simulink model "pokus07_video"  (R2023a)
settings: Solver=VariableStepAuto  StartTime=0.0  StopTime=10.0  RelTol=1e-3
undefined symbols (not defined in the file): c
libraries: Miscellaneous x840, Memory_Blocks_Lib x251, Decoders_Lib x10, simulink_extras x10, Counters_Lib x4, Bit_Multiplexers_Lib x1, Byte_Multiplexers_Lib x1
(part 1 of 5)
settings Model: Creator=Jozko Mrkvicka  LastModifiedBy=Jozko Mrkvicka

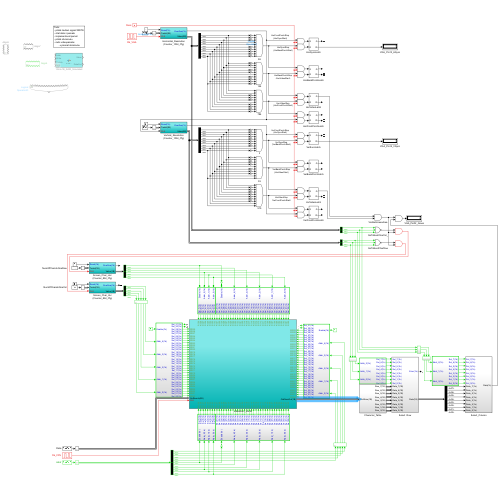
[thumbnail: Simulink's stored preview of the top-level diagram]
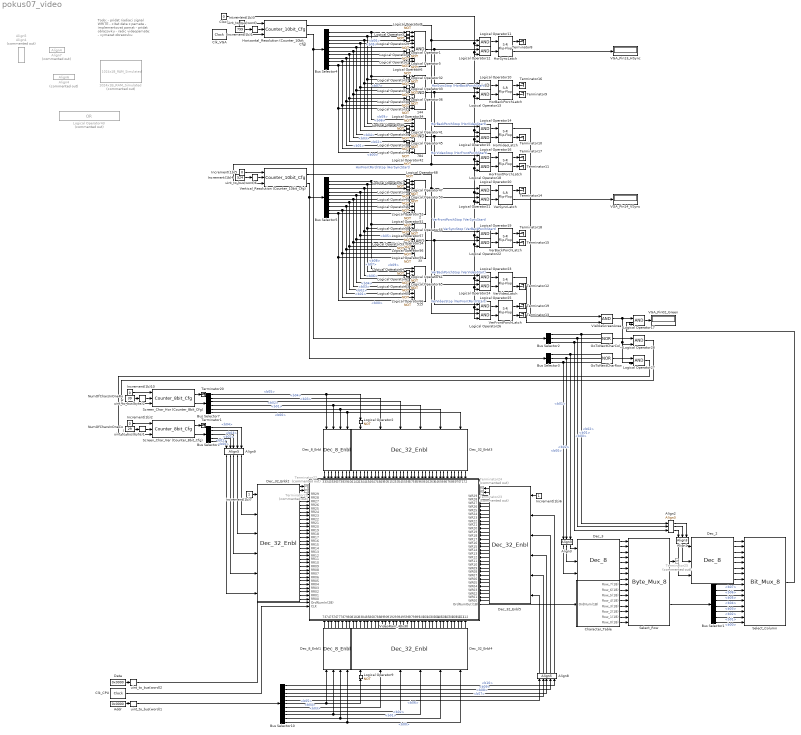
== system pokus07_video ==
  note: Todo:
      | - pridat riadiaci signal WRITE
      | - citat data z pamate
      | - implementovat pamat
      | - pridat obrazovku
      | - radic videopamate:
      | 	- vymazat obrazovku
  1024x1B_RAM_Simulated : Memory_Blocks_Lib/1024x1B_RAM_Simulated  Commented=on  SystemSampleTime=-1  VariantActivationTime=update diagram  Latency=0  AutoFrameSizeCalculation=off
  {2,35,96,144,515,784} (6 alike) : Logic  Inputs=10  IconShape=distinctive  AllPortsSameDT=off  OutDataTypeStr=boolean
  Addr : Constant  Value=0x0000  OutDataTypeStr=uint16
  Align1 : Miscellaneous/Align3  SystemSampleTime=-1  VariantActivationTime=update diagram  Latency=0  AutoFrameSizeCalculation=off
  Align2 : Miscellaneous/Align3  SystemSampleTime=-1  VariantActivationTime=update diagram  Latency=0  AutoFrameSizeCalculation=off
  Align3 : Miscellaneous/Align3  SystemSampleTime=-1  VariantActivationTime=update diagram  Latency=0  AutoFrameSizeCalculation=off
  Align4 : Miscellaneous/Align6  Commented=on
  Align5 : Miscellaneous/Align4  Commented=on
  Align7 : Miscellaneous/Align4  Commented=on
  Align8 : Miscellaneous/Align5
  Align9 : Miscellaneous/Align5
  Bus Selector1 : BusSelector  OutputSignals=b07,b06,b05,b04,b03,b02,b01,b00
  Bus Selector10 : BusSelector  OutputSignals=b10,b09,b08,b07,b06,b05,b04,b03,b02,b01,b00
  Bus Selector2 : BusSelector  OutputSignals=b02,b01,b00
  Bus Selector3 : BusSelector  OutputSignals=b02,b01,b00
  Bus Selector4 : BusSelector  OutputSignals=b09,b08,b07,b06,b05,b04,b03,b02,b01,b00
  Bus Selector5 : BusSelector  OutputSignals=b09,b08,b07,b06,b05,b04,b03,b02,b01,b00
  Bus Selector6 : BusSelector  OutputSignals=b04,b03,b02,b01,b00
  Bus Selector7 : BusSelector  OutputSignals=b05,b04,b03,b02,b01,b00
  Character_Table : Subsystem
  Clk_CPU : simulink_extras/Flip Flops/Clock  period=1
  Clk_VGA : simulink_extras/Flip Flops/Clock  period=1
  Clock : Constant  Value=0  OutDataTypeStr=uint16
  Data : Constant  Value=0x0000  OutDataTypeStr=uint16
  Dec_2 : Decoders_Lib/Dec_8  SystemSampleTime=-1  VariantActivationTime=update diagram  Latency=0  AutoFrameSizeCalculation=off
  Dec_3 : Decoders_Lib/Dec_8  SystemSampleTime=-1  VariantActivationTime=update diagram  Latency=0  AutoFrameSizeCalculation=off
  Dec_32_Enbl{2..5} (4 alike) : Decoders_Lib/Dec_32_Enbl  SystemSampleTime=-1  VariantActivationTime=update diagram  Latency=0  AutoFrameSizeCalculation=off
  Dec_8_Enbl : Decoders_Lib/Dec_8_Enbl  SystemSampleTime=-1  VariantActivationTime=update diagram  Latency=0  AutoFrameSizeCalculation=off
  Dec_8_Enbl1 : Decoders_Lib/Dec_8_Enbl  SystemSampleTime=-1  VariantActivationTime=update diagram  Latency=0  AutoFrameSizeCalculation=off
  GoToNextCharCol_ : Logic  Operator=NOR  Inputs=3  IconShape=distinctive  AllPortsSameDT=off  OutDataTypeStr=boolean
  GoToNextCharRow : Logic  Operator=NOR  Inputs=3  IconShape=distinctive  AllPortsSameDT=off  OutDataTypeStr=boolean
  HorBackPorchLatch : simulink_extras/Flip Flops/S-R Flip-Flop  initial_condition=0
  HorFrontPorchLatch : simulink_extras/Flip Flops/S-R Flip-Flop  initial_condition=0
  HorSyncLatch : simulink_extras/Flip Flops/S-R Flip-Flop  initial_condition=0
  HorVideoLatch : simulink_extras/Flip Flops/S-R Flip-Flop  initial_condition=0
  Horizontal_Resolution (Counter_10bit_Cfg) : Counters_Lib/Counter_10bit_Cfg  SystemSampleTime=-1  VariantActivationTime=update diagram  Latency=0  AutoFrameSizeCalculation=off
  Increment(1b)1 : Constant  Value=799  OutDataTypeStr=uint16
  Increment(1b){2..3,5,10} (4 alike) : Constant  Value=0  OutDataTypeStr=boolean
  Increment(1b)4 : Constant  Value=524  OutDataTypeStr=uint16
  Increment(1b)6 : Constant  OutDataTypeStr=boolean
  Increment(1b)7 : Constant  OutDataTypeStr=boolean
  Logical Operator{1..9,29..42,44..68} (48 alike) : Logic  Operator=NOT  IconShape=distinctive  AllPortsSameDT=off  OutDataTypeStr=boolean
  Logical Operator{10..28} (19 alike) : Logic  IconShape=distinctive  AllPortsSameDT=off  OutDataTypeStr=boolean
  Logical Operator43 : Logic  Commented=on  Operator=OR  Inputs=16  IconShape=distinctive  OutDataTypeStr=boolean
  "NumOfCharsInOneCol      " : Constant  Value=29  OutDataTypeStr=uint8
  "NumOfCharsInOneRow      " : Constant  Value=39  OutDataTypeStr=uint8
  Screen_Char_Hor (Counter_8bit_Cfg) : Counters_Lib/Counter_8bit_Cfg  SystemSampleTime=-1  VariantActivationTime=update diagram  Latency=0  AutoFrameSizeCalculation=off
  Screen_Char_Ver (Counter_8bit_Cfg) : Counters_Lib/Counter_8bit_Cfg  SystemSampleTime=-1  VariantActivationTime=update diagram  Latency=0  AutoFrameSizeCalculation=off
  Select_Column : Bit_Multiplexers_Lib/Bit_Mux_8  SystemSampleTime=-1  VariantActivationTime=update diagram  Latency=0  AutoFrameSizeCalculation=off
  Select_Row : Byte_Multiplexers_Lib/Byte_Mux_8  SystemSampleTime=-1  VariantActivationTime=update diagram  Latency=0  AutoFrameSizeCalculation=off
  Terminator{1,8..20} (14 alike) : Terminator
  Terminator{21..25} (5 alike) : Terminator  Commented=on
  VGA_Pin02_Green : Display
  VGA_Pin13_HSync : Display
  VGA_Pin14_VSync : Display
  VerBackPorchLatch : simulink_extras/Flip Flops/S-R Flip-Flop  initial_condition=0
  VerFrontPorchLatch : simulink_extras/Flip Flops/S-R Flip-Flop  initial_condition=0
  VerSyncLatch : simulink_extras/Flip Flops/S-R Flip-Flop  initial_condition=0
  VerVideoLatch : simulink_extras/Flip Flops/S-R Flip-Flop  initial_condition=0
  Vertical_Resolution (Counter_10bit_Cfg) : Counters_Lib/Counter_10bit_Cfg  SystemSampleTime=-1  VariantActivationTime=update diagram  Latency=0  AutoFrameSizeCalculation=off
  VideoRam_40x30 : Subsystem
      settings: PortSchema="{\"entries\":[{\"content\":{\"sides\":[{\"content\":{\"connectorIds\":[\"In1\",\"In2\",\"In3\",\"In4\",\"In5\",\"In6\",\"In7\",\"In8\",\"In9\",\"In10\",\"In11\",\"In12\",\"In13\",\"In14\",\"In15\",\"In16\",\"In17\",\"In18\",\"In19\",\"In20\",\"In21\",\"In22\",\"In23\",\"In24\",\"In25\",\"In26\",\"In27\",\"In28\",\"In29\",\"In30\",\"In31\",\"In32\"]},\"type\":\"ConnectorPlacement.EquallySpacedRectSide\",\"uuid\":\"d52aabea-5fd3-45ae-978c-84320c8647aa\"},{\"content\":{\"connectorIds\":[\"In113\",\"In114\",\"In115\",\"In116\",\"In117\",\"In118\",\"In119\",\"In120\",\"In121\",\"In122\",\"In123\",\"In124\",\"In125\",\"In126\",\"In127\",\"In128\",\"In129\",\"In130\",\"In131\",\"In132\",\"In133\",\"In134\",\"In135\",\"In136\",\"In137\",\"In138\",\"In139\",\"In140\",\"In141\",\"In142\",\"Out1\"],\"side\":\"RIGHT\"},\"type\":\"ConnectorPlacement.EquallySpacedRectSide\",\"uuid\":\"ee274acf-b359-4074-8e34-ab1b10a37285\"},{\"content\":{\"connectorIds\":[\"In33\",\"In34\",\"In35\",\"In36\",\"In37\",\"In38\",\"In39\",\"In40\",\"In41\",\"In42\",\"In43\",\"In44\",\"In45\",\"In46\",\"In47\",\"In48\",\"In49\",\"In50\",\"In51\",\"In52\",\"In53\",\"In54\",\"In55\",\"In56\",\"In57\",\"In58\",\"In59\",\"In60\",\"In61\",\"In62\",\"In63\",\"In64\",\"In65\",\"In66\",\"In67\",\"In68\",\"In69\",\"In70\",\"In71\",\"In72\"],\"side\":\"TOP\"},\"type\":\"ConnectorPlacement.EquallySpacedRectSide\",\"uuid\":\"3a97b239-3869-4833-a172-72387572f73b\"},{\"content\":{\"connectorIds\":[\"In73\",\"In74\",\"In75\",\"In76\",\"In77\",\"In78\",\"In79\",\"In80\",\"In81\",\"In82\",\"In83\",\"In84\",\"In85\",\"In86\",\"In87\",\"In88\",\"In89\",\"In90\",\"In91\",\"In92\",\"In93\",\"In94\",\"In95\",\"In96\",\"In97\",\"In98\",\"In99\",\"In100\",\"In101\",\"In102\",\"In103\",\"In104\",\"In105\",\"In106\",\"In107\",\"In108\",\"In109\",\"In110\",\"In111\",\"In112\"],\"side\":\"BOTTOM\"},\"type\":\"ConnectorPlacement.EquallySpacedRectSide\",\"uuid\":\"8b58b7b1-bd99-4026-8076-2b8578d087d3\"}]},\"type\":\"ConnectorPlacement.EquallySpacedConnector\",\"uuid\":\"3d92f392-72fb-430c-bd15-19a5abeff511\"}],\"packageUris\":[\"http://schema.mathworks.com/mf0/Connector/R2020b\"],\"version\":\"1.0\"}"
  VisibleScreenArea : Logic  IconShape=distinctive  AllPortsSameDT=off  OutDataTypeStr=boolean
  uint_to_bus(byte)1 : Miscellaneous/uint_to_bus(byte)  SystemSampleTime=-1  VariantActivationTime=update diagram  Latency=0  AutoFrameSizeCalculation=off
  uint_to_bus(byte)2 : Miscellaneous/uint_to_bus(byte)  SystemSampleTime=-1  VariantActivationTime=update diagram  Latency=0  AutoFrameSizeCalculation=off
  uint_to_bus(word){,1..2,6} (4 alike) : Miscellaneous/uint_to_bus(word)
  wires:
  Dec_32_Enbl2/3 -> VideoRam_40x30/1(RR29)
  Dec_32_Enbl2/4 -> VideoRam_40x30/2(RR28)
  Dec_32_Enbl2/5 -> VideoRam_40x30/3(RR27)
  Dec_32_Enbl2/6 -> VideoRam_40x30/4(RR26)
  Dec_32_Enbl2/7 -> VideoRam_40x30/5(RR25)
  Dec_32_Enbl2/8 -> VideoRam_40x30/6(RR24)
  Dec_32_Enbl2/9 -> VideoRam_40x30/7(RR23)
  Dec_32_Enbl2/10 -> VideoRam_40x30/8(RR22)
  Dec_32_Enbl2/11 -> VideoRam_40x30/9(RR21)
  Dec_32_Enbl2/12 -> VideoRam_40x30/10(RR20)
  Dec_32_Enbl2/13 -> VideoRam_40x30/11(RR19)
  Dec_32_Enbl2/14 -> VideoRam_40x30/12(RR18)
  Dec_32_Enbl2/15 -> VideoRam_40x30/13(RR17)
  Dec_32_Enbl2/16 -> VideoRam_40x30/14(RR16)
  Dec_32_Enbl2/17 -> VideoRam_40x30/15(RR15)
  Dec_32_Enbl2/18 -> VideoRam_40x30/16(RR14)
  Dec_32_Enbl2/19 -> VideoRam_40x30/17(RR13)
  Dec_32_Enbl2/20 -> VideoRam_40x30/18(RR12)
  Dec_32_Enbl2/21 -> VideoRam_40x30/19(RR11)
  Dec_32_Enbl2/22 -> VideoRam_40x30/20(RR10)
  Dec_32_Enbl2/23 -> VideoRam_40x30/21(RR09)
  Dec_32_Enbl2/24 -> VideoRam_40x30/22(RR08)
  Dec_32_Enbl2/25 -> VideoRam_40x30/23(RR07)
  Dec_32_Enbl2/26 -> VideoRam_40x30/24(RR06)
  Dec_32_Enbl2/27 -> VideoRam_40x30/25(RR05)
  Dec_32_Enbl2/28 -> VideoRam_40x30/26(RR04)
  Dec_32_Enbl2/29 -> VideoRam_40x30/27(RR03)
  Dec_32_Enbl2/30 -> VideoRam_40x30/28(RR02)
  Dec_32_Enbl2/31 -> VideoRam_40x30/29(RR01)
  Dec_32_Enbl2/32 -> VideoRam_40x30/30(RR00)
  Screen_Char_Ver (Counter_8bit_Cfg)/2 -> Bus Selector6/1
  Screen_Char_Ver (Counter_8bit_Cfg)/1 -> Terminator1/1
  uint_to_bus(byte)1/1 -> Screen_Char_Ver (Counter_8bit_Cfg)/2
  "NumOfCharsInOneCol      "/1 -> uint_to_bus(byte)1/1
  Align9/1 -> Dec_32_Enbl2/6
  Align9/2 -> Dec_32_Enbl2/5
  Align9/3 -> Dec_32_Enbl2/4
  Align9/4 -> Dec_32_Enbl2/3
  Align9/5 -> Dec_32_Enbl2/2
  Increment(1b)7/1 -> Dec_32_Enbl2/1
  Select_Column/1 -> Logical Operator17/2
  Screen_Char_Hor (Counter_8bit_Cfg)/2 -> Bus Selector7/1
  "NumOfCharsInOneRow      "/1 -> uint_to_bus(byte)2/1
  Increment(1b)10/1 -> Screen_Char_Hor (Counter_8bit_Cfg)/1
  Bus Selector7/6 -> Dec_8_Enbl/4, Dec_32_Enbl3/6  "<b00>"
  Bus Selector7/5 -> Dec_8_Enbl/3, Dec_32_Enbl3/5  "<b01>"
  Bus Selector7/4 -> Dec_8_Enbl/2, Dec_32_Enbl3/4  "<b02>"
  Bus Selector7/3 -> Dec_32_Enbl3/3  "<b03>"
  Bus Selector7/2 -> Dec_32_Enbl3/2  "<b04>"
  Bus Selector7/1 -> Dec_8_Enbl/1, Logical Operator2/1  "<b05>"
  Logical Operator2/1 -> Dec_32_Enbl3/1
  Bus Selector6/1 -> Align9/5  "<b04>"
  Bus Selector6/2 -> Align9/4  "<b03>"
  Bus Selector6/3 -> Align9/3  "<b02>"
  Bus Selector6/4 -> Align9/2  "<b01>"
  Bus Selector6/5 -> Align9/1  "<b00>"
  Align3/2 -> Dec_3/2
  Align3/3 -> Dec_3/1
  Align3/1 -> Dec_3/3
  Logical Operator9/1 -> Dec_32_Enbl4/1
  Dec_32_Enbl5/3 -> VideoRam_40x30/113(WR29)
  Dec_32_Enbl5/4 -> VideoRam_40x30/114(WR28)
  Dec_32_Enbl5/5 -> VideoRam_40x30/115(WR27)
  Dec_32_Enbl5/6 -> VideoRam_40x30/116(WR26)
  Dec_32_Enbl5/7 -> VideoRam_40x30/117(WR25)
  Dec_32_Enbl5/8 -> VideoRam_40x30/118(WR24)
  Dec_32_Enbl5/9 -> VideoRam_40x30/119(WR23)
  Dec_32_Enbl5/10 -> VideoRam_40x30/120(WR22)
  Dec_32_Enbl5/11 -> VideoRam_40x30/121(WR21)
  Dec_32_Enbl5/12 -> VideoRam_40x30/122(WR20)
  Dec_32_Enbl5/13 -> VideoRam_40x30/123(WR19)
  Dec_32_Enbl5/14 -> VideoRam_40x30/124(WR18)
  Dec_32_Enbl5/15 -> VideoRam_40x30/125(WR17)
  Dec_32_Enbl5/16 -> VideoRam_40x30/126(WR16)
  Dec_32_Enbl5/17 -> VideoRam_40x30/127(WR15)
  Dec_32_Enbl5/18 -> VideoRam_40x30/128(WR14)
  Dec_32_Enbl5/19 -> VideoRam_40x30/129(WR13)
  Dec_32_Enbl5/20 -> VideoRam_40x30/130(WR12)
  Dec_32_Enbl5/21 -> VideoRam_40x30/131(WR11)
  Dec_32_Enbl5/22 -> VideoRam_40x30/132(WR10)
  Dec_32_Enbl5/23 -> VideoRam_40x30/133(WR09)
  Dec_32_Enbl5/24 -> VideoRam_40x30/134(WR08)
  Dec_32_Enbl5/25 -> VideoRam_40x30/135(WR07)
  Dec_32_Enbl5/26 -> VideoRam_40x30/136(WR06)
  Dec_32_Enbl5/27 -> VideoRam_40x30/137(WR05)
  Dec_32_Enbl5/28 -> VideoRam_40x30/138(WR04)
  Dec_32_Enbl5/29 -> VideoRam_40x30/139(WR03)
  Dec_32_Enbl5/30 -> VideoRam_40x30/140(WR02)
  Dec_32_Enbl5/31 -> VideoRam_40x30/141(WR01)
  Dec_32_Enbl5/32 -> VideoRam_40x30/142(WR00)
  Dec_32_Enbl4/1 -> VideoRam_40x30/81(WC31)
  Dec_32_Enbl4/2 -> VideoRam_40x30/82(WC30)
  Dec_32_Enbl4/3 -> VideoRam_40x30/83(WC29)
  Dec_32_Enbl4/4 -> VideoRam_40x30/84(WC28)
  Dec_32_Enbl4/5 -> VideoRam_40x30/85(WC27)
  Dec_32_Enbl4/6 -> VideoRam_40x30/86(WC26)
  Dec_32_Enbl4/7 -> VideoRam_40x30/87(WC25)
  Dec_32_Enbl4/8 -> VideoRam_40x30/88(WC24)
  Dec_32_Enbl4/9 -> VideoRam_40x30/89(WC23)
  Dec_32_Enbl4/10 -> VideoRam_40x30/90(WC22)
  Dec_32_Enbl4/11 -> VideoRam_40x30/91(WC21)
  Dec_32_Enbl4/12 -> VideoRam_40x30/92(WC20)
  Dec_32_Enbl4/13 -> VideoRam_40x30/93(WC19)
  Dec_32_Enbl4/14 -> VideoRam_40x30/94(WC18)
  Dec_32_Enbl4/15 -> VideoRam_40x30/95(WC17)
  Dec_32_Enbl4/16 -> VideoRam_40x30/96(WC16)
  Dec_32_Enbl4/17 -> VideoRam_40x30/97(WC15)
  Dec_32_Enbl4/18 -> VideoRam_40x30/98(WC14)
  Dec_32_Enbl4/19 -> VideoRam_40x30/99(WC13)
  Dec_32_Enbl4/20 -> VideoRam_40x30/100(WC12)
  Dec_32_Enbl4/21 -> VideoRam_40x30/101(WC11)
  Dec_32_Enbl4/22 -> VideoRam_40x30/102(WC10)
  Dec_32_Enbl4/23 -> VideoRam_40x30/103(WC09)
  Dec_32_Enbl4/24 -> VideoRam_40x30/104(WC08)
  Dec_32_Enbl4/25 -> VideoRam_40x30/105(WC07)
  Dec_32_Enbl4/26 -> VideoRam_40x30/106(WC06)
  Dec_32_Enbl4/27 -> VideoRam_40x30/107(WC05)
  Dec_32_Enbl4/28 -> VideoRam_40x30/108(WC04)
  Dec_32_Enbl4/29 -> VideoRam_40x30/109(WC03)
  Dec_32_Enbl4/30 -> VideoRam_40x30/110(WC02)
  Dec_32_Enbl4/31 -> VideoRam_40x30/111(WC01)
  Dec_32_Enbl4/32 -> VideoRam_40x30/112(WC00)
  Dec_8_Enbl1/8 -> VideoRam_40x30/80(WC32)
  Dec_8_Enbl1/6 -> VideoRam_40x30/78(WC34)
  Dec_8_Enbl1/7 -> VideoRam_40x30/79(WC33)
  Dec_8_Enbl1/2 -> VideoRam_40x30/74(WC38)
  Dec_8_Enbl1/1 -> VideoRam_40x30/73(WC39)
  Dec_8_Enbl1/4 -> VideoRam_40x30/76(WC36)
  Dec_8_Enbl1/5 -> VideoRam_40x30/77(WC35)
  Dec_8_Enbl1/3 -> VideoRam_40x30/75(WC37)
  Addr/1 -> uint_to_bus(word)1/1
  uint_to_bus(word)1/1 -> Bus Selector10/1
  Bus Selector10/11 -> Dec_8_Enbl1/4, Dec_32_Enbl4/6  "<b00>"
  Bus Selector10/10 -> Dec_8_Enbl1/3, Dec_32_Enbl4/5  "<b01>"
  Bus Selector10/9 -> Dec_8_Enbl1/2, Dec_32_Enbl4/4  "<b02>"
  Bus Selector10/8 -> Dec_32_Enbl4/3  "<b03>"
  Bus Selector10/7 -> Dec_32_Enbl4/2  "<b04>"
  Bus Selector10/6 -> Dec_8_Enbl1/1, Logical Operator9/1  "<b05>"
  Bus Selector10/5 -> Align8/1  "<b06>"
  Bus Selector10/4 -> Align8/2  "<b07>"
  Bus Selector10/3 -> Align8/3  "<b08>"
  Bus Selector10/2 -> Align8/4  "<b09>"
  Bus Selector10/1 -> Align8/5  "<b10>"
  Align8/1 -> Dec_32_Enbl5/6
  Align8/2 -> Dec_32_Enbl5/5
  Align8/3 -> Dec_32_Enbl5/4
  Align8/4 -> Dec_32_Enbl5/3
  Align8/5 -> Dec_32_Enbl5/2
  Data/1 -> uint_to_bus(word)2/1
  uint_to_bus(word)2/1 -> VideoRam_40x30/31(OrdNumIn(2B))
  VideoRam_40x30/1(OrdNumOut(1B)) -> Character_Table/1(OrdNum(1B))
  Character_Table/1(Row_7(1B)) -> Select_Row/9
  Character_Table/2(Row_6(1B)) -> Select_Row/10
  Character_Table/3(Row_5(1B)) -> Select_Row/11
  Character_Table/4(Row_4(1B)) -> Select_Row/12
  Character_Table/5(Row_3(1B)) -> Select_Row/13
  Character_Table/6(Row_2(1B)) -> Select_Row/14
  Character_Table/7(Row_1(1B)) -> Select_Row/15
  Character_Table/8(Row_0(1B)) -> Select_Row/16
  Dec_3/1 -> Select_Row/1
  Dec_3/2 -> Select_Row/2
  Dec_3/3 -> Select_Row/3
  Dec_3/4 -> Select_Row/4
  Dec_3/5 -> Select_Row/5
  Dec_3/6 -> Select_Row/6
  Dec_3/7 -> Select_Row/7
  Dec_3/8 -> Select_Row/8
  Select_Row/2 -> Bus Selector1/1
  Bus Selector1/1 -> Select_Column/9  "<b07>"
  Bus Selector1/2 -> Select_Column/10  "<b06>"
  Bus Selector1/3 -> Select_Column/11  "<b05>"
  Bus Selector1/4 -> Select_Column/12  "<b04>"
  Bus Selector1/5 -> Select_Column/13  "<b03>"
  Bus Selector1/6 -> Select_Column/14  "<b02>"
  Bus Selector1/7 -> Select_Column/15  "<b01>"
  Bus Selector1/8 -> Select_Column/16  "<b00>"
  Dec_2/1 -> Select_Column/1
  Dec_2/2 -> Select_Column/2
  Dec_2/3 -> Select_Column/3
  Dec_2/4 -> Select_Column/4
  Dec_2/5 -> Select_Column/5
  Dec_2/6 -> Select_Column/6
  Dec_2/7 -> Select_Column/7
  Dec_2/8 -> Select_Column/8
  Align1/3 -> Dec_2/1
  Align1/2 -> Dec_2/2
  Align1/1 -> Dec_2/3
  Increment(1b)1/1 -> uint_to_bus(word)/1
  uint_to_bus(word)/1 -> Horizontal_Resolution (Counter_10bit_Cfg)/2
  Increment(1b)3/1 -> Horizontal_Resolution (Counter_10bit_Cfg)/1
  Horizontal_Resolution (Counter_10bit_Cfg)/2 -> Bus Selector4/1, Bus Selector2/1
  Horizontal_Resolution (Counter_10bit_Cfg)/1 -> Logical Operator18/1, Vertical_Resolution (Counter_10bit_Cfg)/3, Logical Operator11/1  "HorFrontPorchStop (HorSyncStart)"
  96/1 -> Logical Operator12/1, Logical Operator10/1  "HorSyncStop (HorBackPorchStart)"
  144/1 -> Logical Operator14/1, Logical Operator13/1  "HorBackPorchStop (HorVideoStart)"
  784/1 -> Logical Operator16/1, Logical Operator15/1  "HorVideoStop (HorFrontPorchStart)"
  515/1 -> Logical Operator25/1, Logical Operator24/1  "VerVideoStop (VerFrontPorchStart)"
  Vertical_Resolution (Counter_10bit_Cfg)/2 -> Bus Selector5/1, Bus Selector3/1
  Increment(1b)4/1 -> uint_to_bus(word)6/1
  2/1 -> Logical Operator19/1, Logical Operator21/1  "VerSyncStop (VerBackPorchStart)"
  35/1 -> Logical Operator23/1, Logical Operator22/1  "VerBackPorchStop (VerVideoStart)"
  Vertical_Resolution (Counter_10bit_Cfg)/1 -> Logical Operator20/1, Logical Operator26/1  "VerFrontPorchStop (VerSyncStart)"
  Increment(1b)5/1 -> Vertical_Resolution (Counter_10bit_Cfg)/1
  uint_to_bus(word)6/1 -> Vertical_Resolution (Counter_10bit_Cfg)/2
  Logical Operator11/1 -> HorSyncLatch/1
  Logical Operator12/1 -> HorSyncLatch/2
  Clock/1 -> Logical Operator26/2, Logical Operator25/2, Logical Operator24/2, Logical Operator23/2, Logical Operator22/2, Logical Operator19/2, Logical Operator21/2, Logical Operator20/2, Logical Operator18/2, Logical Operator16/2, Logical Operator15/2, Logical Operator14/2, Logical Operator13/2, Logical Operator10/2, Logical Operator12/2, Logical Operator11/2
  HorSyncLatch/1 -> Terminator8/1
  Logical Operator10/1 -> HorBackPorchLatch/1
  HorBackPorchLatch/2 -> Terminator9/1
  Logical Operator13/1 -> HorBackPorchLatch/2
  Logical Operator14/1 -> HorVideoLatch/1
  HorVideoLatch/2 -> Terminator10/1
  Logical Operator15/1 -> HorVideoLatch/2
  Logical Operator16/1 -> HorFrontPorchLatch/1
  HorFrontPorchLatch/2 -> Terminator11/1
  Logical Operator18/1 -> HorFrontPorchLatch/2
  HorSyncLatch/2 -> VGA_Pin13_HSync/1
  Logical Operator20/1 -> VerSyncLatch/1
  Logical Operator24/1 -> VerVideoLatch/2
  Logical Operator23/1 -> VerVideoLatch/1
  VerBackPorchLatch/2 -> Terminator15/1
  Logical Operator19/1 -> VerBackPorchLatch/1
  VerFrontPorchLatch/2 -> Terminator13/1
  VerSyncLatch/1 -> Terminator14/1
  Logical Operator26/1 -> VerFrontPorchLatch/2
  Logical Operator25/1 -> VerFrontPorchLatch/1
  Logical Operator21/1 -> VerSyncLatch/2
  Logical Operator22/1 -> VerBackPorchLatch/2
  VerVideoLatch/2 -> Terminator12/1
  VerSyncLatch/2 -> VGA_Pin14_VSync/1
  HorVideoLatch/1 -> VisibleScreenArea/1
  VerVideoLatch/1 -> VisibleScreenArea/2
  VisibleScreenArea/1 -> Logical Operator17/1, Logical Operator27/2, Logical Operator28/2
  HorBackPorchLatch/1 -> Terminator16/1
  HorFrontPorchLatch/1 -> Terminator17/1
  VerBackPorchLatch/1 -> Terminator18/1
  VerFrontPorchLatch/1 -> Terminator19/1
  Bus Selector2/1 -> GoToNextCharCol_/1, Align2/1  "<b02>"
  Bus Selector2/2 -> GoToNextCharCol_/2, Align2/2  "<b01>"
  Bus Selector2/3 -> GoToNextCharCol_/3, Align2/3  "<b00>"
  Logical Operator28/1 -> Screen_Char_Hor (Counter_8bit_Cfg)/3
  Logical Operator17/1 -> VGA_Pin02_Green/1
  GoToNextCharCol_/1 -> Logical Operator28/1
  Bus Selector3/1 -> Align3/3, GoToNextCharRow/1  "<b02>"
  Bus Selector3/3 -> Align3/1, GoToNextCharRow/3  "<b00>"
  Bus Selector3/2 -> Align3/2, GoToNextCharRow/2  "<b01>"
  GoToNextCharRow/1 -> Logical Operator27/1
  Logical Operator27/1 -> Screen_Char_Ver (Counter_8bit_Cfg)/3
  Logical Operator4/1 -> 96/6
  Screen_Char_Hor (Counter_8bit_Cfg)/1 -> Terminator20/1
  uint_to_bus(byte)2/1 -> Screen_Char_Hor (Counter_8bit_Cfg)/2
  Increment(1b)2/1 -> Screen_Char_Ver (Counter_8bit_Cfg)/1
  Dec_32_Enbl3/1 -> VideoRam_40x30/41(RC31)
  Dec_32_Enbl3/2 -> VideoRam_40x30/42(RC30)
  Dec_32_Enbl3/3 -> VideoRam_40x30/43(RC29)
  Dec_32_Enbl3/4 -> VideoRam_40x30/44(RC28)
  Dec_32_Enbl3/5 -> VideoRam_40x30/45(RC27)
  Dec_32_Enbl3/6 -> VideoRam_40x30/46(RC26)
  Dec_32_Enbl3/7 -> VideoRam_40x30/47(RC25)
  Dec_32_Enbl3/8 -> VideoRam_40x30/48(RC24)
  Dec_32_Enbl3/9 -> VideoRam_40x30/49(RC23)
  Dec_32_Enbl3/10 -> VideoRam_40x30/50(RC22)
  Dec_32_Enbl3/11 -> VideoRam_40x30/51(RC21)
  Dec_32_Enbl3/12 -> VideoRam_40x30/52(RC20)
  Dec_32_Enbl3/13 -> VideoRam_40x30/53(RC19)
  Dec_32_Enbl3/14 -> VideoRam_40x30/54(RC18)
  Dec_32_Enbl3/15 -> VideoRam_40x30/55(RC17)
  Dec_32_Enbl3/16 -> VideoRam_40x30/56(RC16)
  Dec_32_Enbl3/17 -> VideoRam_40x30/57(RC15)
  Dec_32_Enbl3/18 -> VideoRam_40x30/58(RC14)
  Dec_32_Enbl3/19 -> VideoRam_40x30/59(RC13)
  Dec_32_Enbl3/20 -> VideoRam_40x30/60(RC12)
  Dec_32_Enbl3/21 -> VideoRam_40x30/61(RC11)
  Dec_32_Enbl3/22 -> VideoRam_40x30/62(RC10)
  Dec_32_Enbl3/23 -> VideoRam_40x30/63(RC09)
  Dec_32_Enbl3/24 -> VideoRam_40x30/64(RC08)
  Dec_32_Enbl3/25 -> VideoRam_40x30/65(RC07)
  Dec_32_Enbl3/26 -> VideoRam_40x30/66(RC06)
  Dec_32_Enbl3/27 -> VideoRam_40x30/67(RC05)
  Dec_32_Enbl3/28 -> VideoRam_40x30/68(RC04)
  Dec_32_Enbl3/29 -> VideoRam_40x30/69(RC03)
  Dec_32_Enbl3/30 -> VideoRam_40x30/70(RC02)
  Dec_32_Enbl3/31 -> VideoRam_40x30/71(RC01)
  Dec_32_Enbl3/32 -> VideoRam_40x30/72(RC00)
  Dec_8_Enbl/1 -> VideoRam_40x30/33(RC39)
  Dec_8_Enbl/2 -> VideoRam_40x30/34(RC38)
  Dec_8_Enbl/3 -> VideoRam_40x30/35(RC37)
  Dec_8_Enbl/4 -> VideoRam_40x30/36(RC36)
  Dec_8_Enbl/5 -> VideoRam_40x30/37(RC35)
  Dec_8_Enbl/6 -> VideoRam_40x30/38(RC34)
  Dec_8_Enbl/7 -> VideoRam_40x30/39(RC33)
  Dec_8_Enbl/8 -> VideoRam_40x30/40(RC32)
  Increment(1b)6/1 -> Dec_32_Enbl5/1
  Dec_32_Enbl2/2 -> Terminator21/1
  Dec_32_Enbl2/1 -> Terminator22/1
  Dec_32_Enbl5/2 -> Terminator23/1
  Dec_32_Enbl5/1 -> Terminator24/1
  Select_Row/1 -> Terminator25/1
  Logical Operator7/1 -> 96/8
  Logical Operator6/1 -> 96/9
  Logical Operator5/1 -> 96/10
  Logical Operator1/1 -> 96/7
  Logical Operator29/1 -> 96/3
  Logical Operator3/1 -> 96/2
  Logical Operator8/1 -> 96/1
  Logical Operator34/1 -> 144/10
  Logical Operator36/1 -> 144/8
  Logical Operator32/1 -> 144/2
  Logical Operator31/1 -> 144/4
  Logical Operator30/1 -> 144/7
  Logical Operator33/1 -> 144/5
  Logical Operator37/1 -> 144/1
  Logical Operator35/1 -> 144/9
  Logical Operator42/1 -> 784/10
  Logical Operator45/1 -> 784/8
  Logical Operator38/1 -> 784/7
  Logical Operator41/1 -> 784/5
  Logical Operator44/1 -> 784/9
  Logical Operator40/1 -> 784/3
  Logical Operator39/1 -> 784/4
  Logical Operator49/1 -> 2/5
  Logical Operator47/1 -> 2/4
  Logical Operator50/1 -> 2/6
  Logical Operator51/1 -> 2/10
  Logical Operator46/1 -> 2/7
  Logical Operator52/1 -> 2/8
  Logical Operator48/1 -> 2/3
  Logical Operator56/1 -> 35/6
  Logical Operator54/1 -> 35/4
  Logical Operator53/1 -> 35/7
  Logical Operator59/1 -> 35/8
  Logical Operator55/1 -> 35/3
  Logical Operator63/1 -> 515/5
  Logical Operator61/1 -> 515/4
  Logical Operator64/1 -> 515/2
  Logical Operator65/1 -> 515/6
  Logical Operator60/1 -> 515/7
  Logical Operator66/1 -> 515/8
  Logical Operator62/1 -> 515/3
  Logical Operator68/1 -> 2/1
  Logical Operator67/1 -> 2/2
  Logical Operator57/1 -> 35/2
  Logical Operator58/1 -> 35/1
  Bus Selector4/1 -> 784/1, Logical Operator37/1, Logical Operator8/1  "<b09>"
  Bus Selector4/2 -> 784/2, Logical Operator32/1, Logical Operator3/1  "<b08>"
  Bus Selector4/3 -> Logical Operator40/1, 144/3, Logical Operator29/1  "<b07>"
  Bus Selector4/4 -> Logical Operator39/1, Logical Operator31/1, 96/4  "<b06>"
  Bus Selector4/5 -> Logical Operator41/1, Logical Operator33/1, 96/5  "<b05>"
  Bus Selector4/6 -> Logical Operator4/1, 784/6, 144/6  "<b04>"
  Bus Selector4/7 -> Logical Operator1/1, Logical Operator38/1, Logical Operator30/1  "<b03>"
  Bus Selector4/8 -> Logical Operator7/1, Logical Operator45/1, Logical Operator36/1  "<b02>"
  Bus Selector4/9 -> Logical Operator6/1, Logical Operator44/1, Logical Operator35/1  "<b01>"
  Bus Selector4/10 -> Logical Operator5/1, Logical Operator42/1, Logical Operator34/1  "<b00>"
  Bus Selector5/2 -> Logical Operator67/1, Logical Operator64/1, Logical Operator57/1  "<b08>"
  Bus Selector5/6 -> Logical Operator50/1, Logical Operator56/1, Logical Operator65/1  "<b04>"
  Bus Selector5/1 -> Logical Operator68/1, 515/1, Logical Operator58/1  "<b09>"
  Bus Selector5/5 -> Logical Operator49/1, 35/5, Logical Operator63/1  "<b05>"
  Bus Selector5/4 -> Logical Operator47/1, Logical Operator61/1, Logical Operator54/1  "<b06>"
  Bus Selector5/7 -> Logical Operator46/1, Logical Operator53/1, Logical Operator60/1  "<b03>"
  Bus Selector5/3 -> Logical Operator48/1, Logical Operator55/1, Logical Operator62/1  "<b07>"
  Bus Selector5/9 -> 2/9, 35/9, 515/9  "<b01>"
  Bus Selector5/10 -> Logical Operator51/1, 35/10, 515/10  "<b00>"
  Bus Selector5/8 -> Logical Operator52/1, Logical Operator59/1, Logical Operator66/1  "<b02>"
  Clk_VGA/1 -> Horizontal_Resolution (Counter_10bit_Cfg)/3
  Align2/3 -> Align1/1
  Align2/2 -> Align1/2
  Align2/1 -> Align1/3
  Clk_CPU/1 -> VideoRam_40x30/32(CLK)
